simulink model "linear_model"  (R2023b)
settings: Solver=ode1  StartTime=0.0  StopTime=400  FixedStep=0.01  MaxStep=8.36  RelTol=1e-3
settings Model: Creator=Ali  LastModifiedBy=Ali

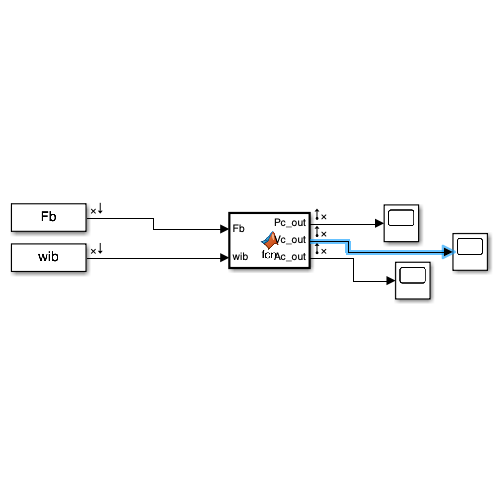
[thumbnail: Simulink's stored preview of the top-level diagram]
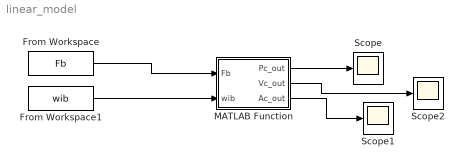
== system linear_model ==
  From Workspace : FromWorkspace  VariableName=Fb
  From Workspace1 : FromWorkspace  VariableName=wib
  MATLAB Function : MATLAB Function  TreatAsAtomicUnit=on
  Scope : Scope
  Scope1 : Scope
  Scope2 : Scope
  wires:
  From Workspace/1 -> MATLAB Function/1(Fb)
  From Workspace1/1 -> MATLAB Function/2(wib)
  MATLAB Function/1(Pc_out) -> Scope/1
  MATLAB Function/3(Ac_out) -> Scope1/1
  MATLAB Function/2(Vc_out) -> Scope2/1

== matlab function linear_model/MATLAB Function ==
  data: Fb input; Pc_out output; wib input; Vc_out output; Ac_out output
function [Pc_out, Vc_out, Ac_out] = fcn(Fb, wib)
%% load data
%% parameters:
%% Sample rate
DeltaT = 0.01; %Sample time
%% Earth Parameters
f = 1/298.2572236;
e = 0.0818191908426;
R0 = 6378137;
ee = e*e;
Omega_e = 7.29211651452621e-5;

%% Initial Conditions
% Initial Position
persistent Pc
if isempty(Pc)
Pc = [0;0;10^4];
end
% Initial Velocity
persistent Vc
if isempty(Vc)
Vc = [-0.0097  200.0138    0.0104]';
end

% Initial Euler Angles

persistent Ac
if isempty(Ac)
Ac = [-0.7771   -0.7770    0.0000]'*10^-6;
end

win = zeros(3, 1);
ADot = zeros(3, 1);
Gn = zeros(3, 1);
VDot = zeros(3, 1);
PDot = zeros(3, 1);


    %% Calculating Force at body frame

    %% Calculating Angular rate at body frame

    %% Calculating Cos transfer Matrix for trasferring  from body frame to navigation frame
    CCLA = cos(Pc(1,1));
    SCLA = sin(Pc(1,1));
    SC2LA = sin(2*Pc(1,1));
    %% Calculating Ground Radious
    RG = R0*(1-f*SCLA*SCLA); %Gussian Radius
    RN = R0*(1-ee)/(1-ee*SCLA*SCLA)^1.5;
    RE = R0/(1-ee*SCLA*SCLA)^0.5;
    %% Sin and Cos Euler Angles
    SCR = sin(Ac(1,1));
    CCR = cos(Ac(1,1));
    SCP = sin(Ac(2,1));
    CCP = cos(Ac(2,1));
    TCP = SCP/CCP;
    %%%%%%%%%%%%%%%%%%%%%%%%%%%%%%%%%%%%%%%%%%%%%%%%%%%%%%%%%%%%%%%%%%%%%%%%%%%
    %%%%%%%%%%%%%%%%%%%%%%%%%%%%%%%%%%%%%%%%%%%%%%%%%%%%%%%%%%%%%%%%%%%%%%%%%%%
    %% Body rate at NED frame from body rate at inertila frame
    win(1,1) = Omega_e*CCLA + Vc(2,1)/(RE+Pc(3,1));
    win(2,1) = -1* Vc(1,1)/(RN+Pc(3,1));
    win(3,1) = -1*Omega_e*SCLA - Vc(2,1)*SCLA/((RE+Pc(3,1))*CCLA);
    %%
    Cbn=CalcCbn(Ac);
    wnb = wib - Cbn' * win;
    %% Calculating new attitude rate from body rate at NED
    ADot(1,1) = wnb(1,1)+(wnb(2,1)*SCR + wnb(3,1)*CCR)*TCP;
    ADot(2,1) = wnb(2,1)*CCR -wnb(3,1)*SCR;
    ADot(3,1) = (wnb(2,1)*SCR+ wnb(3,1)*CCR)/CCP;
    %% Calculating new attitude angles
    Ac = Ac + ADot * DeltaT;
    %% Calculating Cos transfer Matrix for trasferring  from body frame to navigation frame
    %% Velocity Update
    %% Transferring Force from body frame to NED frame
    Fn=Cbn*Fb;
    %% Calculating Gravity vector
    gh0 = 9.780318*(1+5.3024e-3*SCLA*SCLA - 5.9e-6*SC2LA);
    gh = gh0/(1+Pc(3,1)/RG)^2;
    Gn(1,1)=0;
    Gn(2,1)=0;
    Gn(3,1)=gh;
    %% Calculating Vdot
    VDot(1,1)= Vc(1,1)*Vc(3,1)/(RN+Pc(3,1))-Vc(2,1)*Vc(2,1)*SCLA/((RE+Pc(3,1))*CCLA)...
            -2*Omega_e*Vc(2,1)*SCLA;
    VDot(2,1)= 2*Omega_e*Vc(1,1)*SCLA + Vc(1,1)*Vc(2,1)*SCLA/((RE+Pc(3,1))*CCLA)...
            +2*Omega_e*Vc(3,1)*CCLA + Vc(2,1)*Vc(3,1)/(RE+Pc(3,1));
    VDot(3,1)= -2*Omega_e*Vc(2,1)*CCLA - Vc(2,1)*Vc(2,1)/(RE+Pc(3,1))...
            -Vc(1,1)*Vc(1,1)/(RN+Pc(3,1));
    VDot = Fn+VDot+Gn;
    %% Calculating new linear velocity:euler discrtization
    Vc = Vc + VDot*DeltaT;
    %% Position Update:
    PDot(1,1) = Vc(1,1)/(RN+Pc(3,1));
    PDot(2,1) = Vc(2,1)/((RE+Pc(3,1))*CCLA);
    PDot(3,1) = -1 * Vc(3,1);
    %% Calculating new geodetic position
    Pc = Pc+PDot*DeltaT;
    %%
    Pc_out = Pc;
    Vc_out = Vc;
    Ac_out = Ac;
end



% function for calculating Cos transfer Matrix for trasferring  from body frame to navigation frame
function Cbn=CalcCbn(Ac)
    Sphi = sin(Ac(1,1));
    Cphi = cos(Ac(1,1));
    Stheta = sin(Ac(2,1));
    Ctheta = cos(Ac(2,1));
    Cpsi = cos(Ac(3,1));
    Spsi = sin(Ac(3,1));
    Cbn = [Ctheta*Cpsi, Sphi*Stheta*Cpsi-Cphi*Spsi, Cphi*Stheta*Cpsi+Sphi*Spsi;
           Ctheta*Spsi, Sphi*Stheta*Spsi+Cphi*Cpsi, Cphi*Stheta*Spsi-Sphi*Cpsi;
           -1*Stheta, Sphi*Ctheta, Cphi*Ctheta];
end
